simulink model "LoadCell"  (R2024b)
settings: Solver=FixedStepAuto  StartTime=0.0  StopTime=inf  FixedStep=0.01  RelTol=1e-3  EnableMultiTasking=on
libraries: stm32f4xxblockslib x1
settings Model: STM32="{\"AnalogInput\":[{\"ID\":\"Poten1:1\"},{\"ID\":\"LoadCell:1\"}]}"  Creator=pongn  LastModifiedBy=pongn
settings OptimizationCC: DefaultParameterBehavior=Inlined  EnhancedBackFolding=on  PassReuseOutputArgsAs=Individual arguments  ZeroExternalMemoryAtStartup=off  ZeroInternalMemoryAtStartup=off  MaxStackSize=512  OptimizeBlockOrder=speed  DifferentSizesBufferReuse=on  OptimizationCustomize=off  EfficientTunableParamExpr=on
settings DebuggingCC: ParameterTunabilityLossMsg=error
settings HardwareCC: ProdBitPerPointer=32  ProdBitPerSizeT=32  ProdBitPerPtrDiffT=32  ProdLargestAtomicInteger=Long  ProdLargestAtomicFloat=Double  ProdWordSize=32  ProdLongLongMode=on  ProdHWDeviceType=ARM Compatible->ARM Cortex-M
settings SFSimCC: MATLABDynamicMemAlloc=off
settings RTWCC: Description=Embedded Coder  SystemTargetFile=ert.tlc  HardwareBoard=STM32G4xx Based  TemplateMakefile=ert_default_tmf  Toolchain=GNU Tools for ARM Embedded Processors
settings CodeAppCC: ForceParamTrailComments=on  IgnoreCustomStorageClasses=off  OperatorAnnotations=on  SimulinkDataObjDesc=on  SFDataObjDesc=on  InsertBlockDesc=on
settings ERTTargetCC: TargetLangStandard=C99 (ISO)  CodeReplacementLibrary=ARM Cortex-M  ExtModeTransport=3  ExtModeStaticAlloc=on  ExtModeStaticAllocSize=2048  ExtModeMexFile=ext_xcp  ExtModeIntrfLevel=Level2 - Open

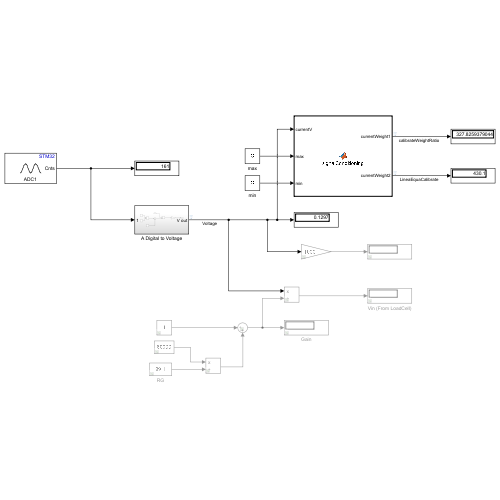
[thumbnail: Simulink's stored preview of the top-level diagram]
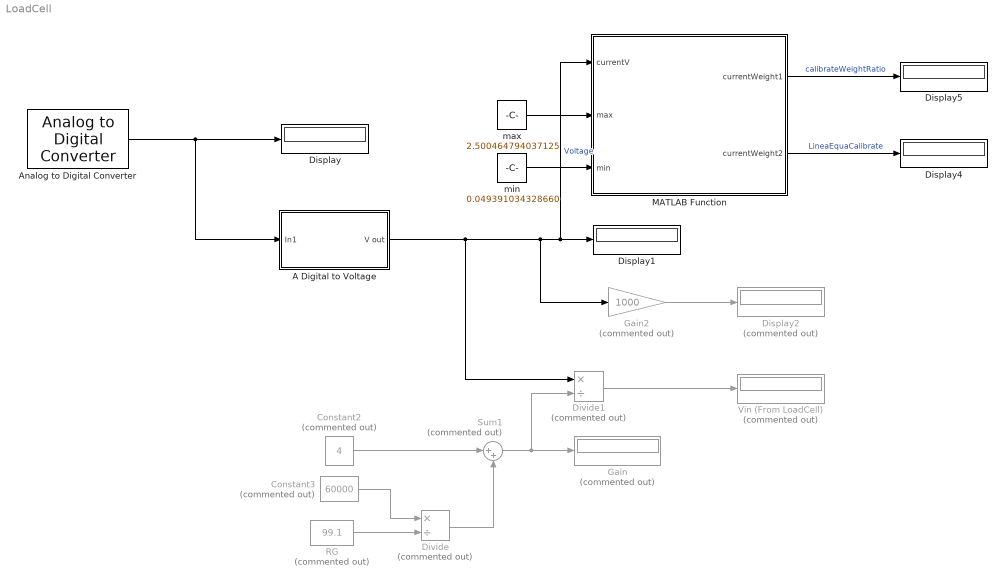
== system LoadCell ==
  A Digital to Voltage : Subsystem
  Analog to Digital Converter : stm32f4xxblockslib/Analog to Digital Converter  ADCModule=ADC1  ConversionGroup=Regular  TriggerMode=Trigger and read  NumberOfConversions=1  EnableBufferConv=off  BufferLength=1  OutputStatus=off  SampleTime=-1  EnableSimPort=off  hoistedMaskSrc=ECSoC/ECSimCodegen/Analog to Digital Converter
  Constant2 : Constant  Commented=on  Value=4
  Constant3 : Constant  Commented=on  Value=60000
  Display{,1,4..5} (4 alike) : Display
  Display2 : Display  Commented=on
  Divide : Product  Commented=on  Inputs=*/
  Divide1 : Product  Commented=on  Inputs=*/
  Gain : Display  Commented=on
  Gain2 : Gain  Commented=on  Gain=1000
  MATLAB Function : MATLAB Function  TreatAsAtomicUnit=on
  RG : Constant  Commented=on  Value=99.1
  Sum1 : Sum  Commented=on  Inputs=|++
  Vin (From LoadCell) : Display  Commented=on
  max : Constant  Value=2.500464794037125
  min : Constant  Value=0.049391034328660
  wires:
  Analog to Digital Converter/1 -> A Digital to Voltage/1(In1), Display/1
  A Digital to Voltage/1(V out) -> MATLAB Function/1(currentV), Display1/1, Gain2/1, Divide1/1  "Voltage"
  Constant2/1 -> Sum1/1
  Divide/1 -> Sum1/2
  Constant3/1 -> Divide/1
  RG/1 -> Divide/2
  MATLAB Function/1(currentWeight1) -> Display5/1  "calibrateWeightRatio"
  Sum1/1 -> Divide1/2, Gain/1
  Divide1/1 -> Vin (From LoadCell)/1
  Gain2/1 -> Display2/1
  max/1 -> MATLAB Function/2(max)
  min/1 -> MATLAB Function/3(min)
  MATLAB Function/2(currentWeight2) -> Display4/1  "LineaEquaCalibrate"

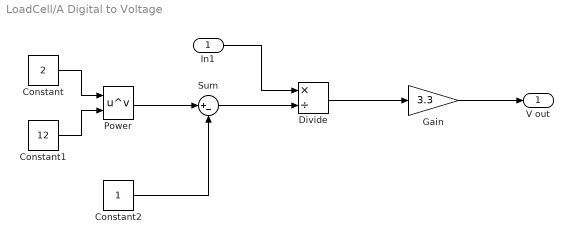
== system LoadCell/A Digital to Voltage ==
  In1 : Inport
  Constant : Constant  Value=2
  Constant1 : Constant  Value=12
  Constant2 : Constant
  Divide : Product  Inputs=*/
  Gain : Gain  Gain=3.3
  Power : Math  Operator=pow
  Sum : Sum  Inputs=|+-
  V out : Outport
  wires:
  Constant/1 -> Power/1
  Constant2/1 -> Sum/2
  Sum/1 -> Divide/2
  Power/1 -> Sum/1
  Divide/1 -> Gain/1
  Constant1/1 -> Power/2
  Gain/1 -> V out/1
  In1/1 -> Divide/1

== matlab function LoadCell/MATLAB Function ==
  data: currentV input; currentWeight1 output; max input; min input; currentWeight2 output
function [currentWeight1,currentWeight2] = signalConditioning(currentV, max, min)
    %Measured 1 : Ratio
    %Measured 2 : Linear Equation
    range = max-min;
    ratio = (currentV-min)/range;
    
    currentWeight1 = ratio * 10000;
    currentWeight2 = (currentV * 4027.34386713426) - 92.3987738807251;
    end
